simulink model "week2_4"  (R2020b)
settings: Solver=VariableStepAuto  StartTime=0.0  StopTime=10.0  RelTol=1e-3
settings Model: Creator=MY lenovo  LastModifiedBy=MY lenovo

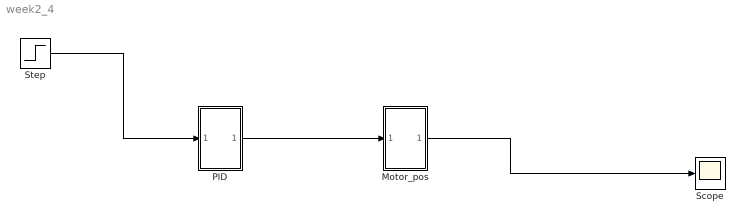
== system week2_4 ==
  Motor_pos : Subsystem
  PID : Subsystem
  Scope : Scope
  Step : Step  SampleTime=0
  wires:
  Motor_pos/1(Out1) -> Scope/1
  Step/1 -> PID/1(Input)
  PID/1(Output) -> Motor_pos/1(In1)

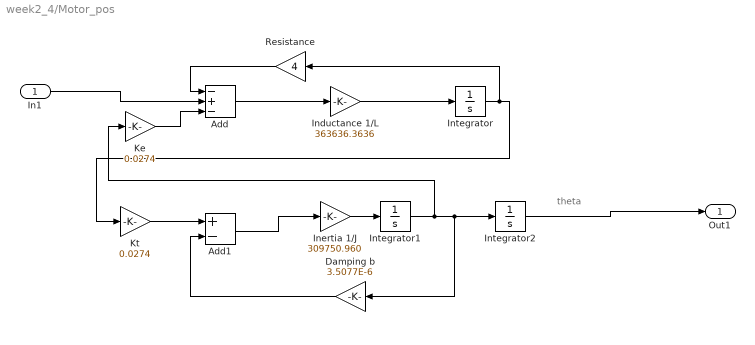
== system week2_4/Motor_pos ==
  note: theta
  In1 : Inport
  Add : Sum  Inputs=-+-
  Add1 : Sum  Inputs=+-
  Damping b : Gain  Gain=3.5077E-6
  Inductance 1/L : Gain  Gain=363636.3636
  Inertia 1/J : Gain  Gain=309750.960
  Integrator : Integrator
  Integrator1 : Integrator
  Integrator2 : Integrator
  Ke : Gain  Gain=0.0274
  Kt : Gain  Gain=0.0274
  Resistance : Gain  Gain=4
  Out1 : Outport
  wires:
  Add/1 -> Inductance 1/L/1
  Resistance/1 -> Add/1
  Kt/1 -> Add1/1
  Inductance 1/L/1 -> Integrator/1
  Ke/1 -> Add/3
  Inertia 1/J/1 -> Integrator1/1
  Integrator/1 -> Resistance/1, Kt/1
  Damping b/1 -> Add1/2
  Integrator1/1 -> Ke/1, Damping b/1, Integrator2/1
  Add1/1 -> Inertia 1/J/1
  Integrator2/1 -> Out1/1
  In1/1 -> Add/2

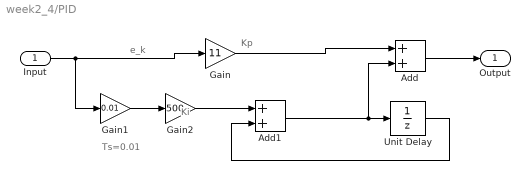
== system week2_4/PID ==
  note: Ts=0.01
  note: Kp
  note: e_k
  note: Ki
  Input : Inport  OutDataTypeStr=double  PortDimensions=1  SampleTime=0
  Add : Sum
  Add1 : Sum
  Gain : Gain  Gain=11
  Gain1 : Gain  Gain=0.01
  Gain2 : Gain  Gain=500
  Unit Delay : UnitDelay  SampleTime=-1  HasFrameUpgradeWarning=on
  Output : Outport  OutDataTypeStr=double  PortDimensions=1  SampleTime=0
  wires:
  Unit Delay/1 -> Add1/2
  Input/1 -> Gain/1, Gain1/1
  Gain2/1 -> Add1/1
  Add1/1 -> Unit Delay/1, Add/2
  Gain/1 -> Add/1
  Gain1/1 -> Gain2/1
  Add/1 -> Output/1
